simulink model "Blockset_Practica_Autosintonizado"  (Simulink 4.0)
settings: Solver=ode45  StartTime=0.0  StopTime=10.0  RelTol=1e-3
undefined symbols (not defined in the file): A, A0, Am, B, Blockset_Practica2, Diseño, nd, nn, ts
libraries: dsparch4 x1, simulink3 x1, dspsrcs4 x1
settings Model: BooleanDataType=on

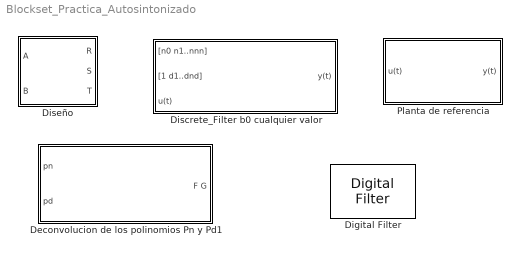
== system Blockset_Practica_Autosintonizado ==
  Deconvolucion de los polinomios Pn y Pd1 : Subsystem  AncestorBlock=Blockset_Practica2/Deconvolucion de los polinomios Pn y Pd1  SimViewingDevice=off
      settings: Permissions=ReadWrite  RTWFcnNameOpts=Auto  RTWFileNameOpts=Auto
      mask Display: disp('Division de los\n  polinomios pn y pd\n  \n [F,G] = deconv (pn,pd)')
  Digital Filter : dsparch4/Digital Filter  TypePopup=IIR (poles & zeros)  IIRFiltStruct=Direct form II transposed  AllPoleFiltStruct=Direct form  FIRFiltStruct=Direct form  CoeffSource=Specify via dialog  NumCoeffs=[1 2]  DenCoeffs=[1 0.1]  BiQuadCoeffs=[1 0.3 0.4 1 0.1 0.2]  LatticeCoeffs=[0.2 0.4]  denIgnore=on  FiltPerSampPopup=One filter per frame  IC=0  ICnum=0  ICden=0
  Discrete_Filter b0 cualquier valor : Subsystem  AncestorBlock=Blockset_Practica2/Discrete_Filter b0 cualquier valor  SimViewingDevice=off  mask{nd=nd, nn=nn, ts=ts}
      mask prompts: nd "Orden del polinomio denominador (nd)"; nn "Orden del polinomio numerador (nn)"; ts "Periodo de muestreo (ts)"
      mask help:
      | Block con comportamiento similar al Discrete Filter de la libreria Discrete.
      | Las entradas son:
      | El vector de coeficientes del numerador (comenzando desde n0)
      | [n0 n1...nnn]
      | El vector de coeficientes del denominador comenzando desde d0=1 polinomio monico) [1 d1...dnd]
      | La excitacion u(t)
      settings: Permissions=ReadWrite  RTWFcnNameOpts=Auto  RTWFileNameOpts=Auto
      mask Display: disp('   DISCRETE FILTER')
  Diseño : Subsystem  AncestorBlock=Blockset_Practica2/Diseño  SimViewingDevice=off  mask{Am=Am, A0=A0}
      settings: Permissions=ReadWrite  RTWFcnNameOpts=Auto  RTWFileNameOpts=Auto
      mask Display: disp('Diseño')
  Planta de referencia : Subsystem  SimViewingDevice=off  mask{A=[1.0000   -0.8500    0.3500   -0.0367], B=[0 0.5300   -0.4], C=[1.0000   -0.875  .15], mean=0, variance=.001, ts=ts}
      mask prompts: A "A(q)"; B "B(q)"; C "C(q)"; mean "Valor medio de e(t)"; variance "Varianza de e(t)"; ts "Tiempo de muestreo"
      settings: Permissions=ReadWrite  RTWFcnNameOpts=Auto  RTWFileNameOpts=Auto
      mask Display: disp(' Planta \n ARMAX')

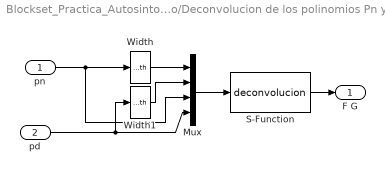
== system Blockset_Practica_Autosintonizado/Deconvolucion de los polinomios Pn y Pd1 ==
  pn : Inport  Port=1  PortDimensions=-1  SampleTime=-1  DataType=auto
      settings: SignalType=auto
  pd : Inport  Port=2  PortDimensions=-1  SampleTime=-1  DataType=auto
      settings: SignalType=auto
  Mux : Mux  Inputs=4
  S-Function : S-Function  FunctionName=deconvolucion  PortCounts=[]  SFunctionModules=''
  Width : Width
  Width1 : Width
  F G : Outport  Port=1
  wires:
  S-Function/1 -> F G/1
  pd/1 -> Mux/4, Width1/1
  pn/1 -> Mux/3, Width/1
  Width1/1 -> Mux/2
  Width/1 -> Mux/1
  Mux/1 -> S-Function/1

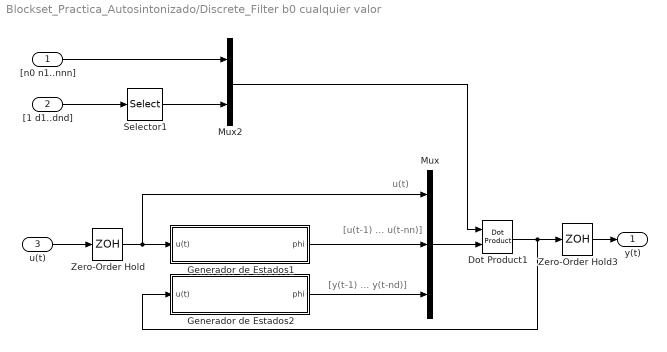
== system Blockset_Practica_Autosintonizado/Discrete_Filter b0 cualquier valor ==
  note: u(t)
  note: [u(t-1) ... u(t-nn)]
  note: [y(t-1) ... y(t-nd)]
  "[n0 n1..nnn]" : Inport  Port=1  PortDimensions=-1  SampleTime=ts  DataType=auto
      settings: SignalType=auto
  "[1 d1..dnd]" : Inport  Port=2  PortDimensions=-1  SampleTime=ts  DataType=auto
      settings: SignalType=auto
  u(t) : Inport  Port=3  PortDimensions=-1  SampleTime=ts  DataType=auto
      settings: SignalType=auto
  Dot Product1 : simulink3/Math/Dot Product
  Generador de Estados1 : Subsystem  SimViewingDevice=off  mask(Generador de Estados){nn=nn, ts=ts}
      mask prompts: nn "Orden del polinomio numerador (nn)"; ts "Periodo de Muestreo"
      mask help: Generador de Estados
      settings: Permissions=ReadWrite  RTWFcnNameOpts=Auto  RTWFileNameOpts=Auto
      mask Help: This block generates the state vector for use with the RLS parameter estimator.
      mask Display: disp('Polinomio Numerador')
  Generador de Estados2 : Subsystem  SimViewingDevice=off  mask(Generador de Estados){nd=nd, ts=ts}
      mask prompts: nd "Orden del polinomio denominador (nd)"; ts "Periodo de Muestreo"
      mask help: Generador de Estados
      settings: Permissions=ReadWrite  RTWFcnNameOpts=Auto  RTWFileNameOpts=Auto
      mask Help: This block generates the state vector for use with the RLS parameter estimator.
      mask Display: disp('Polinomio Denominador')
  Mux : Mux  Inputs=[1 nn nd]
  Mux2 : Mux  Inputs=[nn+1 nd]
  Selector1 : Selector  InputType=Vector  ElementSrc=Internal  Elements=[2:nd+1]  RowSrc=Internal  Rows=1  ColumnSrc=Internal  Columns=1  InputPortWidth=nd+1
  Zero-Order Hold : ZeroOrderHold  SampleTime=ts
  Zero-Order Hold3 : ZeroOrderHold  SampleTime=ts
  y(t) : Outport  Port=1
  wires:
  "[1 d1..dnd]"/1 -> Selector1/1
  Selector1/1 -> Mux2/2
  Mux2/1 -> Dot Product1/1
  "[n0 n1..nnn]"/1 -> Mux2/1
  Generador de Estados2/1(phi) -> Mux/3
  Generador de Estados1/1(phi) -> Mux/2
  Zero-Order Hold/1 -> Mux/1, Generador de Estados1/1(u(t))
  u(t)/1 -> Zero-Order Hold/1
  Dot Product1/1 -> Generador de Estados2/1(u(t)), Zero-Order Hold3/1
  Mux/1 -> Dot Product1/2
  Zero-Order Hold3/1 -> y(t)/1

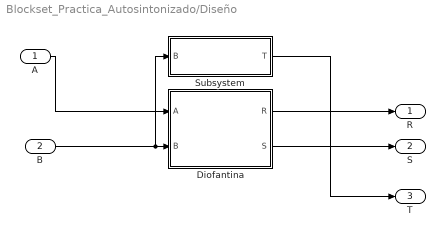
== system Blockset_Practica_Autosintonizado/Diseño ==
  A : Inport  Port=1  PortDimensions=-1  SampleTime=-1  DataType=auto
      settings: SignalType=auto
  B : Inport  Port=2  PortDimensions=-1  SampleTime=-1  DataType=auto
      settings: SignalType=auto
  Diofantina : Subsystem  SimViewingDevice=off  mask{Ac=conv(Am,A0)}
      settings: Permissions=ReadWrite  RTWFcnNameOpts=Auto  RTWFileNameOpts=Auto
      mask Display: disp('Diofantica')
  Subsystem : Subsystem  SimViewingDevice=off  mask{Am=Am, A0=A0}
      settings: Permissions=ReadWrite  RTWFcnNameOpts=Auto  RTWFileNameOpts=Auto
      mask Display: disp('Polinomio T')
  R : Outport  Port=1
  S : Outport  Port=2
  T : Outport  Port=3
  wires:
  B/1 -> Subsystem/1(B), Diofantina/2(B)
  Diofantina/2(S) -> S/1
  A/1 -> Diofantina/1(A)
  Diofantina/1(R) -> R/1
  Subsystem/1(T) -> T/1

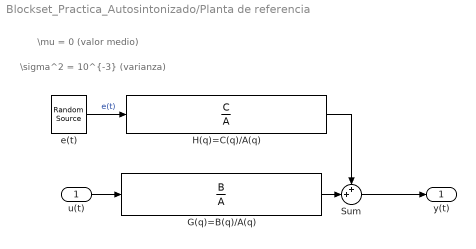
== system Blockset_Practica_Autosintonizado/Planta de referencia ==
  note: \sigma^2 = 10^{-3} (varianza)
  note: \mu = 0 (valor medio)
  u(t) : Inport  Port=1  PortDimensions=-1  SampleTime=-1  DataType=auto
      settings: SignalType=auto
  G(q)=B(q)/A(q) : DiscreteFilter  Numerator=B  Denominator=A  SampleTime=ts  Realization=auto
  H(q)=C(q)/A(q) : DiscreteFilter  Numerator=C  Denominator=A  SampleTime=ts  Realization=auto
  Sum : Sum  Inputs=++|  SaturateOnIntegerOverflow=on
  e(t) : dspsrcs4/Random Source  SrcType=Gaussian  NormMethod=Ziggurat  CltLength=12  Min=0  Max=1  Mean=mean  Var=variance  RepMode=Not repeatable  Seed=1  Inherit=off  SampMode=Discrete  SampTime=ts  SampFrame=1  DataType=Double  OutComplex=Real
  y(t) : Outport  Port=1
  wires:
  H(q)=C(q)/A(q)/1 -> Sum/1
  G(q)=B(q)/A(q)/1 -> Sum/2
  Sum/1 -> y(t)/1
  e(t)/1 -> H(q)=C(q)/A(q)/1  "e(t)"
  u(t)/1 -> G(q)=B(q)/A(q)/1

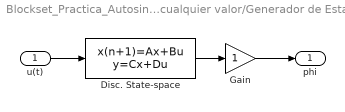
== system Blockset_Practica_Autosintonizado/Discrete_Filter b0 cualquier valor/Generador de Estados1 ==
  u(t) : Inport  Port=1  PortDimensions=-1  SampleTime=-1  DataType=auto
      settings: SignalType=auto
  Disc. State-space : DiscreteStateSpace  A=[zeros(1,nn);eye(nn-1,nn)]  B=[1;zeros(nn-1,1)]  C=eye(nn)  D=[zeros(nn,1)]  X0=0  SampleTime=ts  Realization=auto
  Gain : Gain  Gain=1  Multiplication=Element-wise(K.*u)  SaturateOnIntegerOverflow=on
  phi : Outport  Port=1
  wires:
  Gain/1 -> phi/1
  Disc. State-space/1 -> Gain/1
  u(t)/1 -> Disc. State-space/1

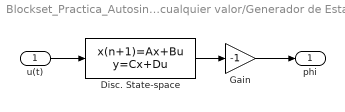
== system Blockset_Practica_Autosintonizado/Discrete_Filter b0 cualquier valor/Generador de Estados2 ==
  u(t) : Inport  Port=1  PortDimensions=-1  SampleTime=-1  DataType=auto
      settings: SignalType=auto
  Disc. State-space : DiscreteStateSpace  A=[zeros(1,nd);eye(nd-1,nd)]  B=[1;zeros(nd-1,1)]  C=eye(nd)  D=[zeros(nd,1)]  X0=0  SampleTime=ts  Realization=auto
  Gain : Gain  Gain=-1  Multiplication=Element-wise(K.*u)  SaturateOnIntegerOverflow=on
  phi : Outport  Port=1
  wires:
  Gain/1 -> phi/1
  Disc. State-space/1 -> Gain/1
  u(t)/1 -> Disc. State-space/1

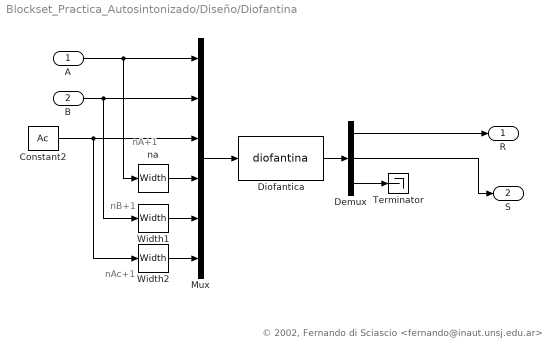
== system Blockset_Practica_Autosintonizado/Diseño/Diofantina ==
  note: © 2002, Fernando di Sciascio <fernando@inaut.unsj.edu.ar>
  note: nB+1
  note: nA+1
  note: nAc+1
  A : Inport  Port=1  PortDimensions=-1  SampleTime=-1  DataType=auto
      settings: SignalType=auto
  B : Inport  Port=2  PortDimensions=-1  SampleTime=-1  DataType=auto
      settings: SignalType=auto
  Constant2 : Constant  Value=Ac
  Demux : Demux  Outputs="[length(Ac)-length(A)+1  length(A)-1  length(A)+length(B)+length(Ac) - (length(Ac)-length(A)+1) -  ( length(A)-1 )+3]"  BusSelectionMode=off
  Diofantica : S-Function  FunctionName=diofantina  PortCounts=[]  SFunctionModules=''
      mask Type: S-function: timestwo
      mask Description: Esta S-function resuelve la ecuacion diofantina
      mask Help:
      | Dados los polinomios A, B, Ac y los ordenes de los polinomios R y S esta
      | S-function resuelve la ecuacion diofantina:
      | 
      |     A*R+B*S=Ac
      mask Display: disp('        Diofantina      ');
  Mux : Mux  Inputs=6
  Terminator : Terminator
  Width1 : Width
  Width2 : Width
  na : Width
  R : Outport  Port=1
  S : Outport  Port=2
  wires:
  Width2/1 -> Mux/6
  Width1/1 -> Mux/5
  na/1 -> Mux/4
  Demux/2 -> S/1
  Demux/1 -> R/1
  B/1 -> Width1/1, Mux/2
  A/1 -> na/1, Mux/1
  Demux/3 -> Terminator/1
  Diofantica/1 -> Demux/1
  Constant2/1 -> Width2/1, Mux/3
  Mux/1 -> Diofantica/1

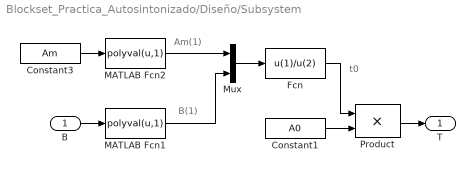
== system Blockset_Practica_Autosintonizado/Diseño/Subsystem ==
  note: t0
  note: Am(1)
  note: B(1)
  B : Inport  Port=1  PortDimensions=-1  SampleTime=-1  DataType=auto
      settings: SignalType=auto
  Constant1 : Constant  Value=A0
  Constant3 : Constant  Value=Am
  Fcn : Fcn  Expr=u(1)/u(2)
  MATLAB Fcn1 : MATLABFcn  MATLABFcn=polyval(u,1)  OutputDimensions=-1  OutputSignalType=auto  Output1D=on
  MATLAB Fcn2 : MATLABFcn  MATLABFcn=polyval(u,1)  OutputDimensions=-1  OutputSignalType=auto  Output1D=on
  Mux : Mux  Inputs=2
  Product : Product  Inputs=2  Multiplication=Element-wise(.*)  SaturateOnIntegerOverflow=on
  T : Outport  Port=1
  wires:
  Constant1/1 -> Product/2
  B/1 -> MATLAB Fcn1/1
  Product/1 -> T/1
  Constant3/1 -> MATLAB Fcn2/1
  Fcn/1 -> Product/1
  MATLAB Fcn1/1 -> Mux/2
  MATLAB Fcn2/1 -> Mux/1
  Mux/1 -> Fcn/1
